simulink model "mytest"  (R2021a)
settings: Solver=FixedStepAuto  StartTime=0.0  StopTime=stopTime  FixedStep=0.01  RelTol=1e-3
values from neighbouring files (symbols this model uses):
  initVal = 5.6    [srdce.m]    (also in tlak.m = pFilter(tLvzorka))
  stepTime = 150    [srdce.m]    (also in tlak.m = 133)
settings Model: Creator=marko  LastModifiedBy=marko

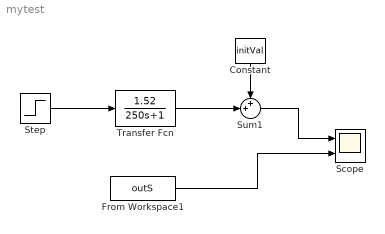
== system mytest ==
  Constant : Constant  Value=initVal
  From Workspace1 : FromWorkspace  VariableName=outS  Interpolate=off  OutputAfterFinalValue=Holding final value
  Scope : Scope  NumInputPorts=2
  Step : Step  Time=stepTime  After=-1  SampleTime=0
  Sum1 : Sum  Inputs=++|
  Transfer Fcn : TransferFcn  Numerator=[1.52]  Denominator=[250 1]
  wires:
  Step/1 -> Transfer Fcn/1
  From Workspace1/1 -> Scope/2
  Constant/1 -> Sum1/1
  Transfer Fcn/1 -> Sum1/2
  Sum1/1 -> Scope/1
